simulink model "lookupTableDynamic_TestGen16"  (R2017b)
settings: Solver=FixedStepDiscrete  StartTime=0.0  StopTime=10.0  RelTol=1e-3
undefined symbols (not defined in the file): Block_TestLib, trigger
libraries: simulink x1
settings Model: Creator=ktrinh  LastModifiedBy=ktrinh
settings DebuggingCC: ParameterOverflowMsg=none

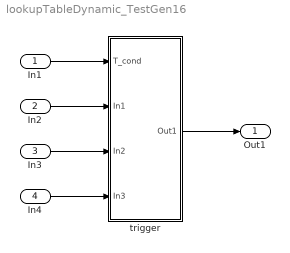
== system lookupTableDynamic_TestGen16 ==
  In1 : Inport
  In2 : Inport  Port=2
  In3 : Inport  Port=3
  In4 : Inport  Port=4
  trigger : Subsystem  AncestorBlock=Block_TestLib/trigger
  Out1 : Outport
  wires:
  In1/1 -> trigger/1(T_cond)
  In2/1 -> trigger/2(In1)
  In3/1 -> trigger/3(In2)
  In4/1 -> trigger/4(In3)
  trigger/1(Out1) -> Out1/1

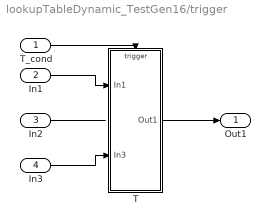
== system lookupTableDynamic_TestGen16/trigger ==
  T_cond : Inport  OutDataTypeStr=boolean
  In1 : Inport  Port=2
  In2 : Inport  Port=3
  In3 : Inport  Port=4
  T : Subsystem  TreatAsAtomicUnit=on
  Out1 : Outport
  wires:
  T_cond/1 -> T/Trigger
  In1/1 -> T/1(In1)
  In2/1 -> ?
  In3/1 -> T/2(In3)
  T/1(Out1) -> Out1/1

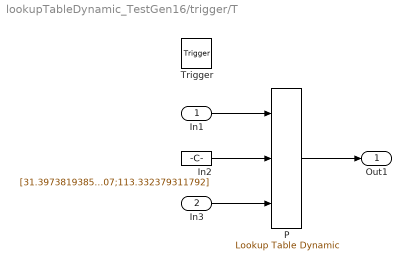
== system lookupTableDynamic_TestGen16/trigger/T ==
  In1 : Inport  OutMin=29.3974  OutMax=115  OutDataTypeStr=uint32  PortDimensions=1
  In3 : Inport  Port=2  PortDimensions=5
  Trigger : TriggerPort  VariantControl=Variant
  In2 : Constant  Value=[31.3973819385122;69.5368453671046;79.8086229552916;103.962607235907;113.332379311792]  OutDataTypeStr=uint32
  P : simulink/Lookup Tables/Lookup Table Dynamic  LookUpMeth=Interpolation-Use End Values  OutDataType=fixdt('int32')  OutScaling=[]  OutputDataTypeScalingMode=Specify via dialog  OutDataTypeStr=int32  DoSatur=off
      settings: SourceProductName=Simulink
  Out1 : Outport
  wires:
  In1/1 -> P/1
  In2/1 -> P/2
  In3/1 -> P/3
  P/1 -> Out1/1
